simulink model "bounce"  (Simulink 7.5)
settings: Solver=ode45  StartTime=0.0  StopTime=10.0  RelTol=1e-3
settings Model: Creator=lab1  LastModifiedBy=lab1

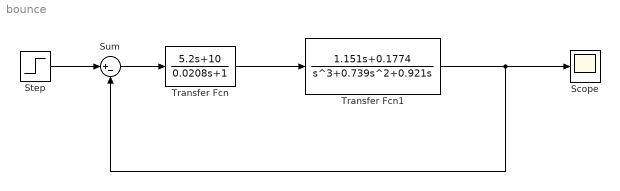
== system bounce ==
  Scope : Scope
  Step : Step  Time=0.01  SampleTime=0
  Sum : Sum  Inputs=|+-  OutDataType=fixdt(1, 16)  OutScaling=2^0
  Transfer Fcn : TransferFcn  Numerator=[5.2 10]  Denominator=[0.0208 1]
  Transfer Fcn1 : TransferFcn  Numerator=[1.151 0.1774]  Denominator=[1 0.739 0.921 0]
  wires:
  Transfer Fcn/1 -> Transfer Fcn1/1
  Sum/1 -> Transfer Fcn/1
  Step/1 -> Sum/1
  Transfer Fcn1/1 -> Scope/1, Sum/2
